simulink model "MassSpringMod_harness"  (R2023b)
settings: Solver=VariableStepAuto  StartTime=0.0  StopTime=100  RelTol=1e-3
settings Model: Creator=20181234  LastModifiedBy=20181234

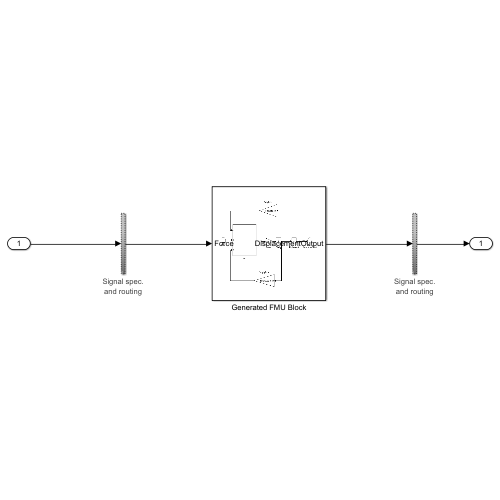
[thumbnail: Simulink's stored preview of the top-level diagram]
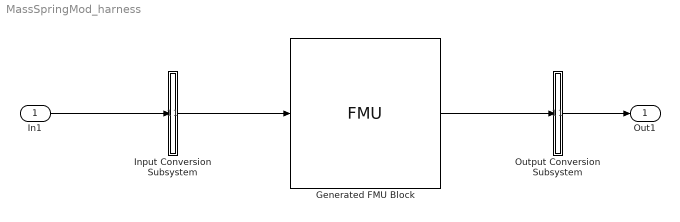
== system MassSpringMod_harness ==
  In1 : Inport  OutDataTypeStr=double  PortDimensions=[1]  SampleTime=1
  Generated FMU Block : FMU  FMUName=MassSpringMod  FMUMode=CoSimulation  FMUSampleTime=1  FMUCreateBusObject=off  FMUInitializeEnumObject=off  dampingCoefficient=-100  mass=5  springConstant=-10  mask(MassSpringMod [Co-Simulation, v2.0]){}
      mask Display:
      | if (exist([Simulink.fileGenControl('get','CacheFolder') '\slprj\_fmu\350ca0e0ac92e0a0f6481d51586bb0f8\MassSpringMod\model.png'],'file'))
      |     image([Simulink.fileGenControl('get','CacheFolder') '\slprj\_fmu\350ca0e0ac92e0a0f6481d51586bb0f8\MassSpringMod\model.png']);
      | else
      |     disp('MassSpringMod');
      | end
      | port_label('output',1,'DisplacementOutput');
      | port_label('input',1,'Force');
  Input Conversion Subsystem : Subsystem  Tag=__SLT_ICS__  Description=|
      | Signal spec.
      | and routing
      settings: AttributesFormatString=%<Description>
  Output Conversion Subsystem : Subsystem  Tag=__SLT_OCS__  Description=|
      | Signal spec.
      | and routing
      settings: AttributesFormatString=%<Description>
  Out1 : Outport
  wires:
  In1/1 -> Input Conversion Subsystem/1(Inport_1)
  Output Conversion Subsystem/1(Outport_1) -> Out1/1
  Input Conversion Subsystem/1(Outport_1) -> Generated FMU Block/1
  Generated FMU Block/1 -> Output Conversion Subsystem/1(Inport_1)

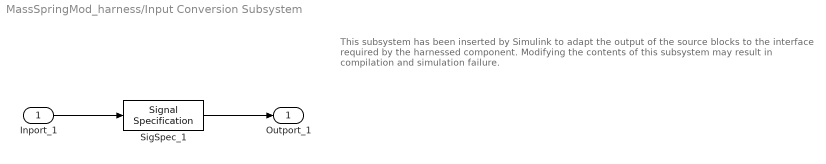
== system MassSpringMod_harness/Input Conversion Subsystem ==
  note: This subsystem has been inserted by Simulink to adapt the output of the source blocks to the interface required by the harnessed component.
      |  Modifying the contents of this subsystem may result in compilation and simulation failure.
  Inport_1 : Inport
  SigSpec_1 : SignalSpecification  OutDataTypeStr=double  Dimensions=[1]  SampleTime=1
  Outport_1 : Outport
  wires:
  SigSpec_1/1 -> Outport_1/1
  Inport_1/1 -> SigSpec_1/1

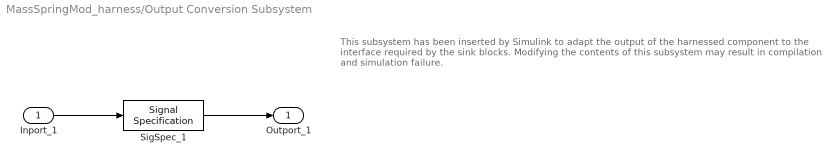
== system MassSpringMod_harness/Output Conversion Subsystem ==
  note: This subsystem has been inserted by Simulink to adapt the output of the harnessed component to the interface required by the sink blocks.
      |  Modifying the contents of this subsystem may result in compilation and simulation failure.
  Inport_1 : Inport
  SigSpec_1 : SignalSpecification  OutDataTypeStr=double  Dimensions=[1]  SampleTime=1
  Outport_1 : Outport
  wires:
  Inport_1/1 -> SigSpec_1/1
  SigSpec_1/1 -> Outport_1/1
